simulink model "Part2_3"  (R2022a)
settings: Solver=VariableStepAuto  StartTime=0.0  StopTime=1000  RelTol=1e-3
values from neighbouring files (symbols this model uses):
  D = diag([0.01, 0.01, 0.01])    [driver2.m]    (also in driver2_2.m; driver2_3.m; driver_2_2.m)
  g = [0,0,-9.81]    [driver2.m]    (also in driver2_2.m; driver2_3.m; driver_2_2.m)
  In = inv(I)    [driver2.m]    (also in driver2_2.m; driver2_3.m; driver_2_2.m)
  k = 0.01    [driver2.m]    (also in driver2_2.m; driver2_3.m; driver_2_2.m)
  m = 0.5    [driver2.m]    (also in driver2_2.m; driver2_3.m; driver_2_2.m)
  tau = [L*k*(Omega(1)^2 - Omega(3)^2) ... (first row only)    [driver2.m]    (also in driver2_2.m; driver2_3.m = 2*w0*[L*k*(Omega(1) - Omega(3)); driver_2_2.m)
  w0 = sqrt(9.81*m/(4*k))    [driver2_3.m]
settings Model: Creator=askeo  LastModifiedBy=askeo

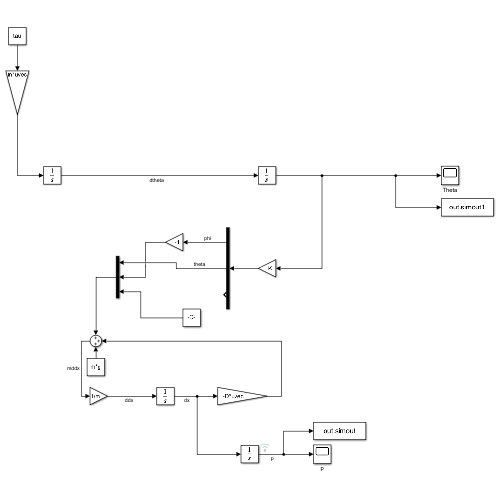
[thumbnail: Simulink's stored preview of the top-level diagram]
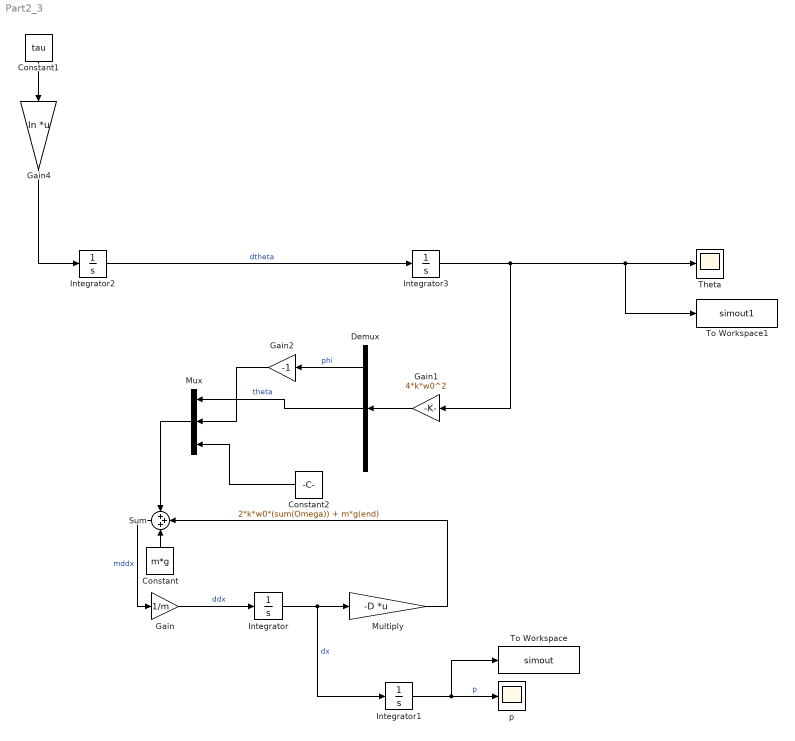
== system Part2_3 ==
  Constant : Constant  Value=m*g
  Constant1 : Constant  Value=tau
  Constant2 : Constant  Value=2*k*w0*(sum(Omega)) + m*g(end)  VectorParams1D=off
  Demux : Demux  Outputs=3
  Gain : Gain  Gain=1/m
  Gain1 : Gain  Gain=4*k*w0^2
  Gain2 : Gain  Gain=-1
  Gain4 : Gain  Gain=In  Multiplication=Matrix(K*u) (u vector)
  Integrator : Integrator  InitialCondition=[0;0;0]
  Integrator1 : Integrator  InitialCondition=[0;0;0]
  Integrator2 : Integrator  InitialCondition=[0;0;0]
  Integrator3 : Integrator  InitialCondition=[0; 0; 0]
  Multiply : Gain  Gain=-D  Multiplication=Matrix(K*u) (u vector)
  Mux : Mux  Inputs=3
  Sum : Sum  Inputs=+++
  Theta : Scope
  To Workspace : ToWorkspace  VariableName=simout  SaveFormat=Timeseries  SampleTime=-1
  To Workspace1 : ToWorkspace  VariableName=simout1  SaveFormat=Timeseries  SampleTime=-1
  p : Scope
  wires:
  Integrator/1 -> Integrator1/1, Multiply/1  "dx"
  Integrator3/1 -> Gain1/1, To Workspace1/1, Theta/1
  Integrator1/1 -> To Workspace/1, p/1  "p"
  Gain4/1 -> Integrator2/1
  Gain/1 -> Integrator/1  "ddx"
  Constant/1 -> Sum/3
  Sum/1 -> Gain/1  "mddx"
  Constant1/1 -> Gain4/1
  Multiply/1 -> Sum/2
  Integrator2/1 -> Integrator3/1  "dtheta"
  Gain1/1 -> Demux/1
  Demux/1 -> Gain2/1  "phi"
  Constant2/1 -> Mux/3
  Mux/1 -> Sum/1
  Gain2/1 -> Mux/2
  Demux/2 -> Mux/1  "theta"
